simulink model "problem2"  (R2020b)
settings: Solver=VariableStepAuto  StartTime=0.0  StopTime=Inf  RelTol=1e-3
settings Model: EnablePacing=on  PacingRate=0.100000  Creator=Lenovo  LastModifiedBy=Admin

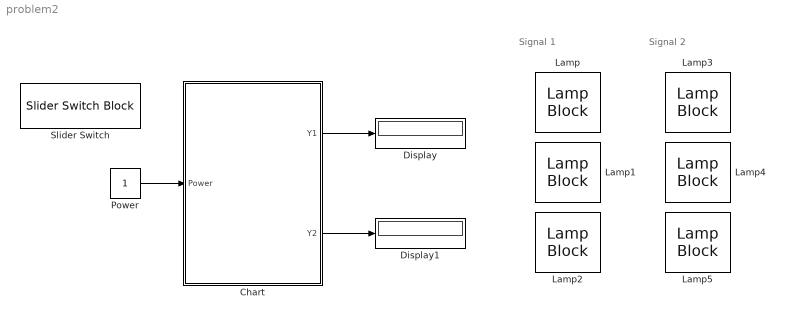
== system problem2 ==
  note: Signal 1
  note: Signal 2
  Chart : Stateflow chart  TreatAsAtomicUnit=on
  Display : Display
  Display1 : Display
  Lamp{,1..5} (6 alike) : LampBlock
  Power : Constant
  Slider Switch : SliderSwitchBlock
      settings: Values={{'Off', 'On'}, [0 1]}
  wires:
  Power/1 -> Chart/1(Power)
  Chart/1(Y1) -> Display/1
  Chart/2(Y2) -> Display1/1

== stateflow chart problem2/Chart ==
  state Signal_ON
    state Stop
      en:
      Y1=0;
      Y2=2;
    state Ready_to_go1
      en:
      Y1=0;
      Y2=2;
    state GO1
      en:
      Y1=1;
      Y2=0;
    state Ready_to_go
      en:
      Y1=2;
      Y2=1;
    state GO
      en:
      Y1=2;
      Y2=0;
    (default) -> Stop
    Ready_to_go1 -> GO1 : {after(5,sec)}
    Stop -> Ready_to_go1 : {after(3,sec)}
    Ready_to_go -> Stop : {after(3,sec)}
    GO1 -> GO : {after(3,sec)}
    GO -> Ready_to_go : {after(5,sec)}
  state Signal_OFF
    en:
    Y1=1;
    Y2=1;
  (default) -> Signal_OFF
  Signal_OFF -> Signal_ON : [Power==1]
  Signal_ON -> Signal_OFF : [Power==0]
  data: Power input; Y1 output; Y2 output
